simulink model "SG__MDL"  (R2022b)
settings: Solver=FixedStepAuto  StartTime=0.0  StopTime=Inf  FixedStep=ts  RelTol=1e-3  EnableMultiTasking=on
model workspace (MAT data in the model file):
  N_trig = Simulink.Parameter
  N_trig.Value = 4
  N_trig.Description = 'number of samples for triggered pulse for recording'
  N_trig.DataType = 'auto'
  N_trig.Complexity = 'real'
  N_trig.Dimensions = [1 1]
  Sig = Simulink.Signal
  Sig.DataType = 'auto'
  Sig.Dimensions = -1
  Sig.DimensionsMode = 'auto'
  Sig.Complexity = 'auto'
  Sig.SampleTime = -1
  Sig.SamplingMode = 'auto'
  dtf_a = Simulink.Parameter
  dtf_a.Value = [1  1  1; 1  1  1; 1  1  1; 1  1  1; 1  1  1; 1  1  1; 1  1  1; 1  1  1; 1  1  1; 1  1  1; 1  1  1; 1  1  1; 1  1  1; 1  1  1; 1  1  1; 1  1  1]
  dtf_a.DataType = 'auto'
  dtf_a.Complexity = 'real'
  dtf_a.Dimensions = [16 3]
  dtf_b = Simulink.Parameter
  dtf_b.Value = [0.5  0.5  0.5; 0.5  0.5  0.5; 0.5  0.5  0.5; 0.5  0.5  0.5; 0.5  0.5  0.5; 0.5  0.5  0.5; 0.5  0.5  0.5; 0.5  0.5  0.5; 0.5  0.5  0.5; 0.5  0.5  0.5; 0.5  0.5  0.5; 0.5  0.5  0.5; 0.5  0.5  0.5; 0.5  0.5  0.5; 0.5  0.5  0.5; 0.5  0.5  0.5]
  dtf_b.DataType = 'auto'
  dtf_b.Complexity = 'real'
  dtf_b.Dimensions = [16 3]
  enable_source = Simulink.Parameter
  enable_source.Value = 0
  enable_source.DataType = 'boolean'
  enable_source.Complexity = 'real'
  enable_source.Dimensions = [1 1]
  freq_fin = Simulink.Parameter
  freq_fin.Value = 1200
  freq_fin.DataType = 'auto'
  freq_fin.Complexity = 'real'
  freq_fin.Dimensions = [1 1]
  freq_ini = Simulink.Parameter
  freq_ini.Value = 150
  freq_ini.DataType = 'auto'
  freq_ini.Complexity = 'real'
  freq_ini.Dimensions = [1 1]
  k_L = Simulink.Parameter
  k_L.Value = [0; 0; 0; 0; 0; 0; 0; 0; 0; 0; 0; 0; 0; 0; 0; 0]
  k_L.Description = 'Coupling on left of ER. [Linear, NL]'
  k_L.DataType = 'auto'
  k_L.Complexity = 'real'
  k_L.Dimensions = [16 1]
  k_L_NL = Simulink.Parameter
  k_L_NL.Value = [0; 0; 0; 0; 0; 0; 0; 0; 0; 0; 0; 0; 0; 0; 0; 0]
  k_L_NL.Description = 'Coupling on left of ER. [Linear, NL]'
  k_L_NL.DataType = 'auto'
  k_L_NL.Complexity = 'real'
  k_L_NL.Dimensions = [16 1]
  k_O_NL = Simulink.Parameter
  k_O_NL.Value = [0; 0; 0; 0; 0; 0; 0; 0; 0; 0; 0; 0; 0; 0; 0; 0]
  k_O_NL.Description = 'Onsite nonlinearity'
  k_O_NL.DataType = 'auto'
  k_O_NL.Complexity = 'real'
  k_O_NL.Dimensions = [16 1]
  k_R = Simulink.Parameter
  k_R.Value = [0; 0; 0; 0; 0; 0; 0; 0; 0; 0; 0; 0; 0; 0; 0; 0]
  k_R.Description = 'Coupling on right of ER. [Linear, NL]'
  k_R.DataType = 'auto'
  k_R.Complexity = 'real'
  k_R.Dimensions = [16 1]
  k_R_NL = Simulink.Parameter
  k_R_NL.Value = [0; 0; 0; 0; 0; 0; 0; 0; 0; 0; 0; 0; 0; 0; 0; 0]
  k_R_NL.Description = 'Coupling on right of ER. [Linear, NL]'
  k_R_NL.DataType = 'auto'
  k_R_NL.Complexity = 'real'
  k_R_NL.Dimensions = [16 1]
  rec = Simulink.Parameter
  rec.Value = 1
  rec.DataType = 'boolean'
  rec.Complexity = 'real'
  rec.Dimensions = [1 1]
  src_select = Simulink.Parameter
  src_select.Value = 0
  src_select.DataType = 'auto'
  src_select.Complexity = 'real'
  src_select.Dimensions = [1 1]
  sweep_gain = Simulink.Parameter
  sweep_gain.Value = 0.02
  sweep_gain.DataType = 'auto'
  sweep_gain.Complexity = 'real'
  sweep_gain.Dimensions = [1 1]
  tmax = Simulink.Parameter
  tmax.Value = 10
  tmax.DataType = 'auto'
  tmax.Complexity = 'real'
  tmax.Dimensions = [1 1]
  ts_rec = Simulink.Parameter
  ts_rec.Value = 0.0001
  ts_rec.DataType = 'auto'
  ts_rec.Complexity = 'real'
  ts_rec.Dimensions = [1 1]
values from neighbouring files (symbols this model uses):
  ts = 400e-6    (= 0.0004)    [StartScript.m]
libraries: simulink x4, dspsrcs4 x2, hdlsllib x2, dspsigattribs x1, dspsigops x1, slrealtimeloglib x1
settings Model: SimulationMode=external  ExplicitPartitioning=on  DataflowThreadingImplementation=Pthreads  Creator=padlewsk  LastModifiedBy=padlewsk
settings SolverCC: AllowMultiTaskInputOutput=on  ConcurrentTasks=on  AlgebraicLoopSolver=TrustRegion  PositivePriorityOrder=on  AutoInsertRateTranBlk=on
settings DataIOCC: SaveFormat=StructureWithTime
settings OptimizationCC: GainParamInheritBuiltInType=on  RollThreshold=33  EfficientFloat2IntCast=on  SimCompilerOptimization=on
settings DebuggingCC: TasksWithSamePriorityMsg=none  UnconnectedInputMsg=warning  UnconnectedOutputMsg=warning  UnconnectedLineMsg=warning  ModelReferenceSymbolNameMessage=none
settings HardwareCC: ProdBitPerLong=64  ProdLongLongMode=on  ProdHWDeviceType=Intel->x86-64 (Linux 64)
settings ModelReferenceCC: EnableRefExpFcnMdlSchedulingChecks=on
settings RTWCC: Description=Simulink Real-Time  SystemTargetFile=slrealtime.tlc  TemplateMakefile=slrealtime_default_tmf  Toolchain=Simulink Real-Time Toolchain  BuildConfiguration=Faster Runs  CodeExecutionProfiling=on  TargetLang=C++
settings SimulinkRealTimeTargetCC: UseGCCFastMath=on

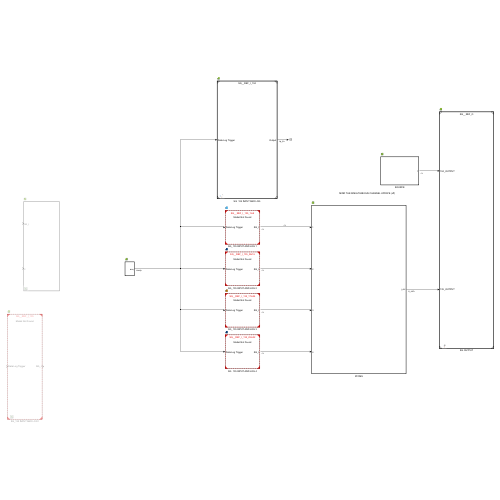
[thumbnail: Simulink's stored preview of the top-level diagram]
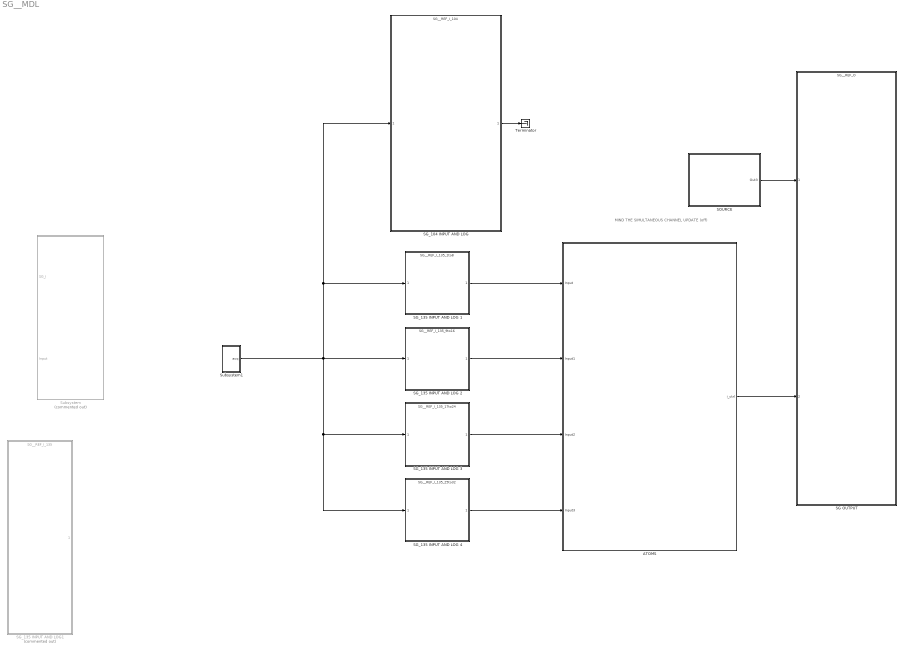
== system SG__MDL ==
  note: MIND THE SIMULTANEOUS CHANNEL UPDATE (off)
  ATOMS : Subsystem  TreatAsAtomicUnit=on
  SG OUTPUT : ModelReference  ModelNameDialog=SG__REF_O.slx  SimulationMode=Normal  ModelReferenceVersion=6.311
  SG_104 INPUT AND LOG : ModelReference  ModelNameDialog=SG__REF_I_104.slx  SimulationMode=Normal  ModelReferenceVersion=6.314
  SG_135 INPUT AND LOG 1 : ModelReference  ModelNameDialog=SG__REF_I_135_1to8.slx  SimulationMode=Normal  ModelReferenceVersion=6.293
  SG_135 INPUT AND LOG 2 : ModelReference  ModelNameDialog=SG__REF_I_135_9to16.slx  SimulationMode=Normal  ModelReferenceVersion=6.294
  SG_135 INPUT AND LOG 3 : ModelReference  ModelNameDialog=SG__REF_I_135_17to24.slx  SimulationMode=Normal  ModelReferenceVersion=6.296
  SG_135 INPUT AND LOG 4 : ModelReference  ModelNameDialog=SG__REF_I_135_25to32.slx  SimulationMode=Normal  ModelReferenceVersion=6.296
  SG_135 INPUT AND LOG1 : ModelReference  Commented=on  ModelNameDialog=SG__REF_I_135.slx  SimulationMode=Normal  ModelReferenceVersion=6.288
  SOURCE : Subsystem  TreatAsAtomicUnit=on
  Subsystem : Subsystem  Commented=on  TreatAsAtomicUnit=on
  Subsystem1 : Subsystem  TreatAsAtomicUnit=on
  Terminator : Terminator
  wires:
  SOURCE/1(Out3) -> SG OUTPUT/1
  SG_135 INPUT AND LOG 1/1 -> ATOMS/1(Input)
  ATOMS/1(i_ctrl) -> SG OUTPUT/2
  SG_104 INPUT AND LOG/1 -> Terminator/1
  Subsystem1/1(acq) -> SG_104 INPUT AND LOG/1, SG_135 INPUT AND LOG 1/1, SG_135 INPUT AND LOG 4/1, SG_135 INPUT AND LOG 3/1, SG_135 INPUT AND LOG 2/1
  SG_135 INPUT AND LOG 2/1 -> ATOMS/2(Input1)
  SG_135 INPUT AND LOG 3/1 -> ATOMS/3(Input2)
  SG_135 INPUT AND LOG 4/1 -> ATOMS/4(Input3)

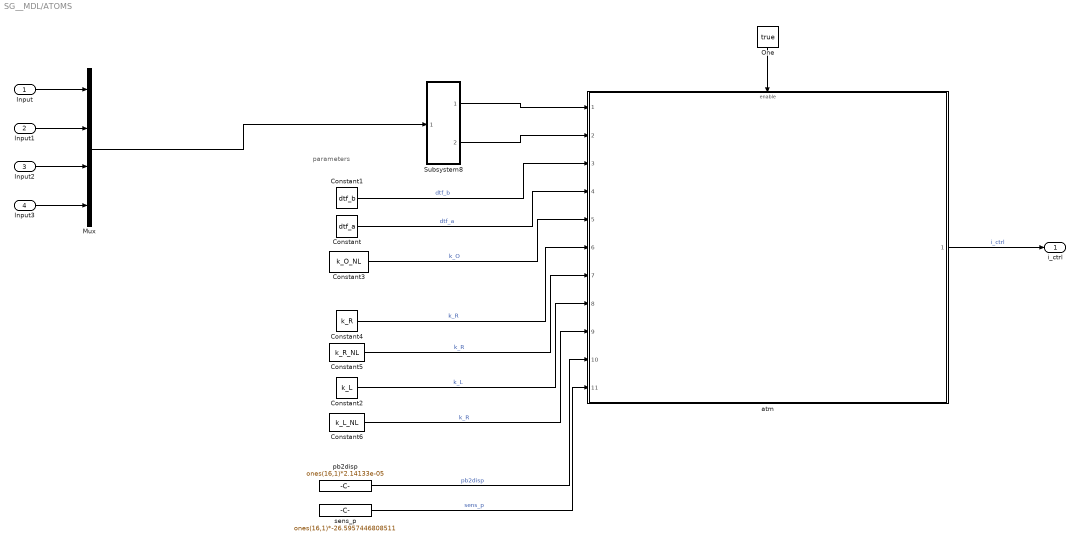
== system SG__MDL/ATOMS ==
  note: parameters
  Input : Inport
  Input1 : Inport  Port=2
  Input2 : Inport  Port=3
  Input3 : Inport  Port=4
  Constant : Constant  Value=dtf_a  SampleTime=-1
  Constant1 : Constant  Value=dtf_b  SampleTime=-1
  Constant2 : Constant  Value=k_L  SampleTime=-1
  Constant3 : Constant  Value=k_O_NL  SampleTime=-1
  Constant4 : Constant  Value=k_R  SampleTime=-1
  Constant5 : Constant  Value=k_R_NL  SampleTime=-1
  Constant6 : Constant  Value=k_L_NL  SampleTime=-1
  Mux : Mux
  One : Constant  Value=true  OutDataTypeStr=Inherit: Inherit via back propagation
  Subsystem8 : Subsystem
  atm : Subsystem  ReferencedSubsystem=atm
  pb2disp : Constant  Value=ones(16,1)*2.14133e-05  SampleTime=-1
  sens_p : Constant  Value=ones(16,1)*-26.5957446808511  SampleTime=-1
  i_ctrl : Outport
  wires:
  One/1 -> atm/Enable
  atm/1 -> i_ctrl/1  "i_ctrl"
  Constant1/1 -> atm/3  "dtf_b"
  Constant/1 -> atm/4  "dtf_a"
  Constant3/1 -> atm/5  "k_O"
  Constant4/1 -> atm/6  "k_R"
  Constant5/1 -> atm/7  "k_R"
  Constant2/1 -> atm/8  "k_L"
  Constant6/1 -> atm/9  "k_R"
  sens_p/1 -> atm/11  "sens_p"
  pb2disp/1 -> atm/10  "pb2disp"
  Subsystem8/2(Input1) -> atm/2
  Subsystem8/1(Input) -> atm/1
  Input/1 -> Mux/1
  Input1/1 -> Mux/2
  Input2/1 -> Mux/3
  Input3/1 -> Mux/4
  Mux/1 -> Subsystem8/1(SG_I)

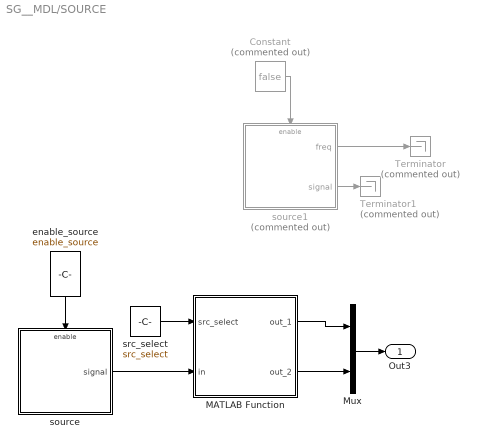
== system SG__MDL/SOURCE ==
  Constant : Constant  Commented=on  Value=false
  MATLAB Function : MATLAB Function  TreatAsAtomicUnit=on
  Mux : Mux  Inputs=2
  Terminator : Terminator  Commented=on
  Terminator1 : Terminator  Commented=on
  enable_source : Constant  Value=enable_source  SampleTime=-1
  source : Subsystem  TreatAsAtomicUnit=on
  source1 : Subsystem  Commented=on  TreatAsAtomicUnit=on
  src_select : Constant  Value=src_select
  Out3 : Outport
  wires:
  Mux/1 -> Out3/1
  Constant/1 -> source1/Enable
  source/1(signal) -> MATLAB Function/2(in)
  src_select/1 -> MATLAB Function/1(src_select)
  MATLAB Function/2(out_2) -> Mux/2
  enable_source/1 -> source/Enable
  source1/2(signal) -> Terminator1/1
  MATLAB Function/1(out_1) -> Mux/1
  source1/1(freq) -> Terminator/1

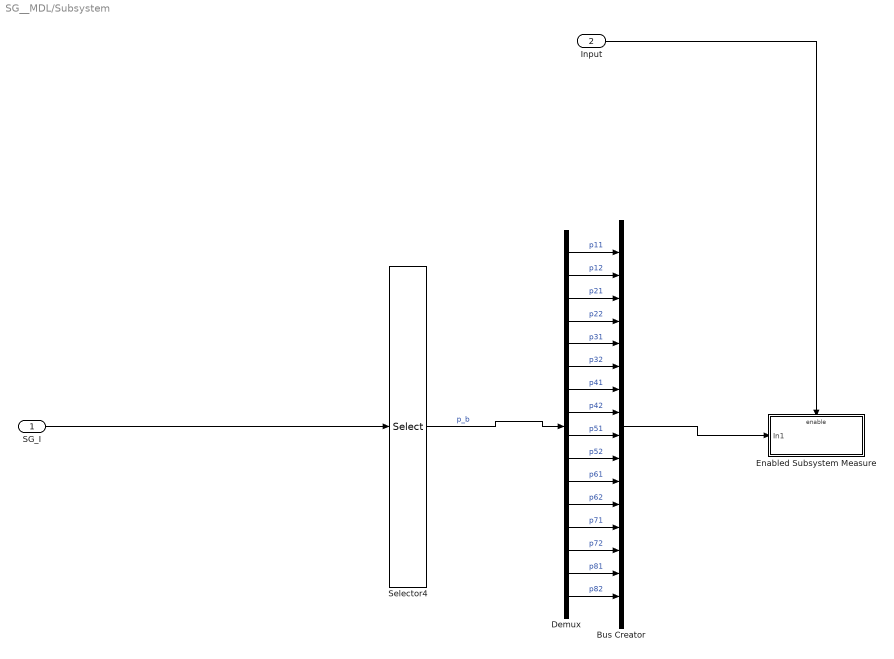
== system SG__MDL/Subsystem ==
  SG_I : Inport  SampleTime=ts
  Input : Inport  Port=2  OutDataTypeStr=boolean
  Bus Creator : BusCreator  Inputs=16
  Demux : Demux  Outputs=16
  Enabled Subsystem Measure : Subsystem
  Selector4 : Selector  InputPortWidth=32  IndexOptions=Index vector (dialog)  Indices=[1:2:32]  OutputSizes=1
  wires:
  Demux/15 -> Bus Creator/15  "p81"
  Bus Creator/1 -> Enabled Subsystem Measure/1(In1)
  Demux/9 -> Bus Creator/9  "p51"
  Demux/12 -> Bus Creator/12  "p62"
  Demux/1 -> Bus Creator/1  "p11"
  Demux/16 -> Bus Creator/16  "p82"
  Demux/8 -> Bus Creator/8  "p42"
  Demux/11 -> Bus Creator/11  "p61"
  Demux/2 -> Bus Creator/2  "p12"
  Demux/7 -> Bus Creator/7  "p41"
  Demux/10 -> Bus Creator/10  "p52"
  Demux/5 -> Bus Creator/5  "p31"
  Demux/13 -> Bus Creator/13  "p71"
  Demux/14 -> Bus Creator/14  "p72"
  Demux/4 -> Bus Creator/4  "p22"
  Demux/6 -> Bus Creator/6  "p32"
  Demux/3 -> Bus Creator/3  "p21"
  Selector4/1 -> Demux/1  "p_b"
  SG_I/1 -> Selector4/1
  Input/1 -> Enabled Subsystem Measure/Enable

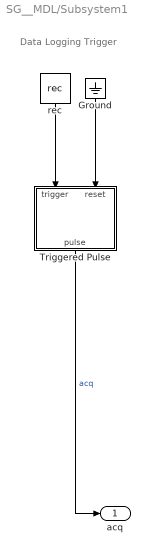
== system SG__MDL/Subsystem1 ==
  note: Data Logging Trigger
  Ground : Ground
  "Triggered Pulse " : Subsystem  TreatAsAtomicUnit=on  mask(Triggered Pulse){N=10/ts}
      mask prompts: N "Length (N samples)"
      mask help: Generates a single pulse of N samples length
  rec : Constant  Value=rec  SampleTime=-1
  acq : Outport  OutDataTypeStr=boolean
  wires:
  Ground/1 -> "Triggered Pulse "/2(reset)
  rec/1 -> "Triggered Pulse "/1(trigger)
  "Triggered Pulse "/1(pulse) -> acq/1  "acq"

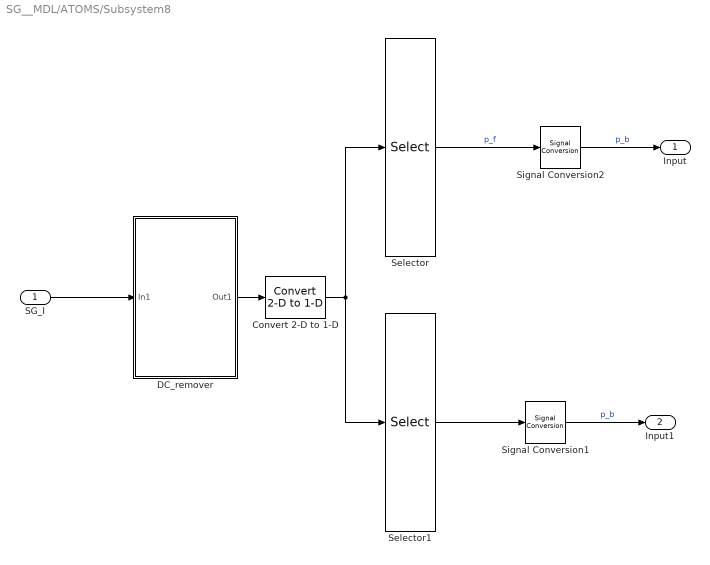
== system SG__MDL/ATOMS/Subsystem8 ==
  SG_I : Inport
  Convert 2-D to 1-D : dspsigattribs/Convert 2-D to 1-D
  DC_remover : Subsystem  TreatAsAtomicUnit=on
      settings: RTWSystemCode=Nonreusable function
  Selector : Selector  InputPortWidth=32  IndexOptions=Index vector (dialog)  Indices=1:2:32  OutputSizes=1
  Selector1 : Selector  InputPortWidth=32  IndexOptions=Index vector (dialog)  Indices=2:2:32  OutputSizes=1
  Signal Conversion1 : SignalConversion  OverrideOpt=off
  Signal Conversion2 : SignalConversion  OverrideOpt=off
  Input : Outport
  Input1 : Outport  Port=2
  wires:
  SG_I/1 -> DC_remover/1(In1)
  Selector1/1 -> Signal Conversion1/1
  DC_remover/1(Out1) -> Convert 2-D to 1-D/1
  Selector/1 -> Signal Conversion2/1  "p_f"
  Signal Conversion1/1 -> Input1/1  "p_b"
  Signal Conversion2/1 -> Input/1  "p_b"
  Convert 2-D to 1-D/1 -> Selector/1, Selector1/1

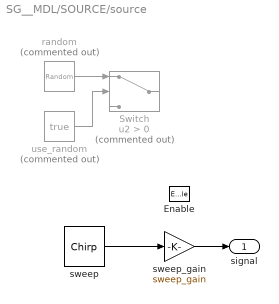
== system SG__MDL/SOURCE/source ==
  Enable : EnablePort  StatesWhenEnabling=reset
  Switch : Switch  Commented=on  Criteria=u2 > Threshold  SaturateOnIntegerOverflow=off  InputSameDT=off
  random : RandomNumber  Commented=on  Variance=0.5  SampleTime=3.5e-05
  sweep : dspsrcs4/Chirp  sweep=Logarithmic  mode=Bidirectional  f0=freq_ini  f1=freq_fin  t1=tmax*2  Tsweep=tmax*2  phase=0  Ts=ts_rec*0 + ts  spf=1  datatype=Double  OutputFrames=off
  sweep_gain : Gain  Gain=sweep_gain
  use_random : Constant  Commented=on  Value=true  SampleTime=-1
  signal : Outport  OutputWhenDisabled=reset  InitialOutput=0  VectorParamsAs1DForOutWhenUnconnected=off
  wires:
  use_random/1 -> Switch/2
  random/1 -> Switch/1
  sweep/1 -> sweep_gain/1
  sweep_gain/1 -> signal/1

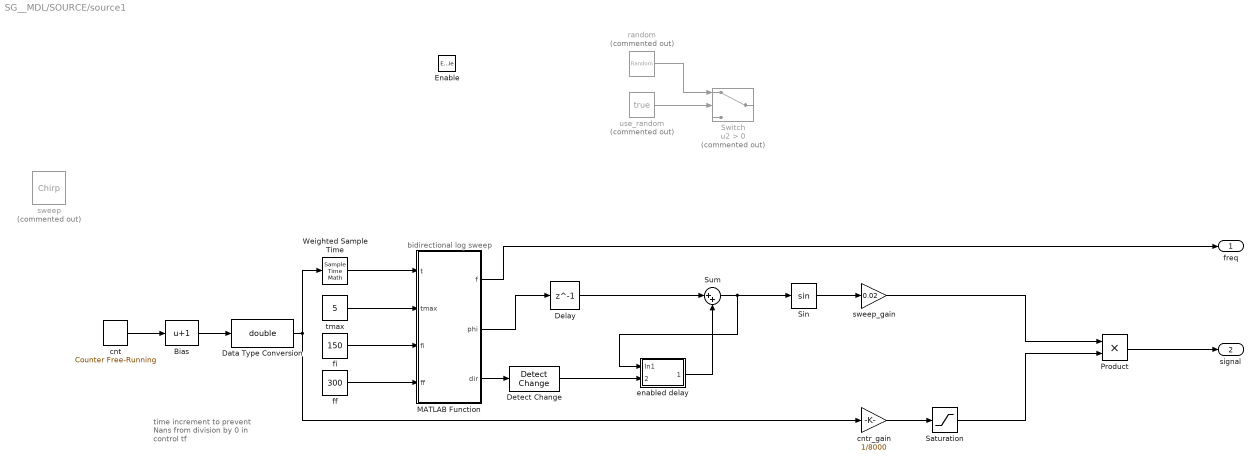
== system SG__MDL/SOURCE/source1 ==
  note: bidirectional log sweep
  note: time increment to prevent Nans from division by 0 in control tf
  Enable : EnablePort  StatesWhenEnabling=reset
  Bias : Bias  Bias=1  SaturateOnIntegerOverflow=off
  Data Type Conversion : DataTypeConversion  OutDataTypeStr=double  SaturateOnIntegerOverflow=off  RndMeth=Floor
  Delay : Delay  DelayLength=1
  Detect Change : simulink/Logic and Bit Operations/Detect Change  vinit=false  OutDataTypeStr=boolean
  MATLAB Function : MATLAB Function  TreatAsAtomicUnit=on
  Product : Product
  Saturation : Saturate  UpperLimit=1  LowerLimit=0
  Sin : Trigonometry
  Sum : Sum  Inputs=|++
  Switch : Switch  Commented=on  Criteria=u2 > Threshold  SaturateOnIntegerOverflow=off  InputSameDT=off
  Weighted Sample Time : SampleTimeMath  TsampMathOp=*
  cnt : simulink/Sources/Counter Free-Running  NumBits=32  tsamp=-1
  cntr_gain : Gain  Gain=1/8000  ParamDataTypeStr=double
  enabled delay : Subsystem
  ff : Constant  Value=300
  fi : Constant  Value=150
  random : RandomNumber  Commented=on  Variance=0.5  SampleTime=3.5e-05
  sweep : dspsrcs4/Chirp  Commented=on  sweep=Logarithmic  mode=Bidirectional  f0=150  f1=1200  t1=10  Tsweep=20  phase=0  Ts=3.5e-05  spf=1  datatype=Double  OutputFrames=off
  sweep_gain : Gain  Gain=0.02
  tmax : Constant  Value=5
  use_random : Constant  Commented=on  Value=true  SampleTime=-1
  freq : Outport  OutputWhenDisabled=reset  InitialOutput=0  VectorParamsAs1DForOutWhenUnconnected=off
  signal : Outport  Port=2  OutputWhenDisabled=reset  InitialOutput=0  VectorParamsAs1DForOutWhenUnconnected=off
  wires:
  use_random/1 -> Switch/2
  random/1 -> Switch/1
  sweep_gain/1 -> Product/1
  cntr_gain/1 -> Saturation/1
  Product/1 -> signal/1
  MATLAB Function/2(phi) -> Delay/1
  Saturation/1 -> Product/2
  Weighted Sample Time/1 -> MATLAB Function/1(t)
  Data Type Conversion/1 -> cntr_gain/1, Weighted Sample Time/1
  MATLAB Function/1(f) -> freq/1
  Sin/1 -> sweep_gain/1
  MATLAB Function/3(dir) -> Detect Change/1
  Detect Change/1 -> enabled delay/2(enable)
  Delay/1 -> Sum/1
  enabled delay/1(Out1) -> Sum/2
  Sum/1 -> enabled delay/1(In1), Sin/1
  cnt/1 -> Bias/1
  Bias/1 -> Data Type Conversion/1
  ff/1 -> MATLAB Function/4(ff)
  tmax/1 -> MATLAB Function/2(tmax)
  fi/1 -> MATLAB Function/3(fi)

== system SG__MDL/Subsystem/Enabled Subsystem Measure ==
  In1 : Inport
  Enable : EnablePort
  File Log : slrealtimeloglib/File Log  decimation=1  inputProcessing=Elements as channels (sample based)
  wires:
  In1/1 -> File Log/1

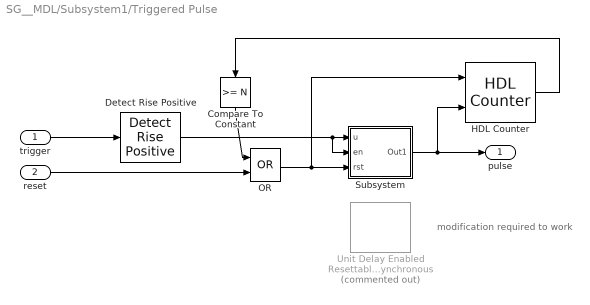
== system SG__MDL/Subsystem1/Triggered Pulse  ==
  note: modification required to work
  trigger : Inport
  reset : Inport  Port=2
  Compare To Constant : simulink/Logic and Bit Operations/Compare To Constant  relop=>=  const=N  OutDataTypeStr=boolean
  Detect Rise Positive : simulink/Logic and Bit Operations/Detect Rise Positive  vinit=0  OutDataTypeStr=boolean
  HDL Counter : hdlsllib/Sources/HDL Counter  CountType=Free running  CountInit=1  CountStep=1  CountMax=25  CountFromType=Initial value  CountFrom=1  CountResetPort=on  CountLoadPort=off  CountEnbPort=on  CountDirPort=off  CountHitOutputPort=off  CountDataType=Unsigned  CountWordLen=32  CountFracLen=0  CountSampTime=1
  OR : Logic  Operator=OR  AllPortsSameDT=off  OutDataTypeStr=boolean
  Subsystem : Subsystem
  Unit Delay Enabled Resettable Synchronous : hdlsllib/Discrete/Unit Delay Enabled Resettable Synchronous  Commented=on  InitialCondition=0.0  SampleTime=-1
  pulse : Outport  VectorParamsAs1DForOutWhenUnconnected=off
  wires:
  OR/1 -> Subsystem/3(rst), HDL Counter/1
  trigger/1 -> Detect Rise Positive/1
  Subsystem/1(Out1) -> HDL Counter/2, pulse/1
  Compare To Constant/1 -> OR/1
  reset/1 -> OR/2
  Detect Rise Positive/1 -> Subsystem/2(en), Subsystem/1(u)
  HDL Counter/1 -> Compare To Constant/1

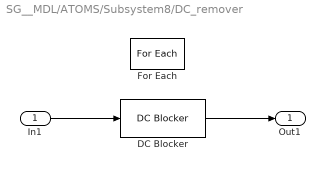
== system SG__MDL/ATOMS/Subsystem8/DC_remover ==
  In1 : Inport  Partition=on  PartitionDimension=1  PartitionWidth=1  PartitionOffset=0
  DC Blocker : dspsigops/DC Blocker  Algorithm=FIR  NormalizedBandwidth=0.001  Length=20  Order=6  SimulateUsing=Code generation
      settings: LibrarySourceBlock=dsphdlsupportsigops/DC Blocker
  For Each : ForEach  DisableCoverage=on
  Out1 : Outport  ConcatenationDimension=1
  wires:
  In1/1 -> DC Blocker/1
  DC Blocker/1 -> Out1/1

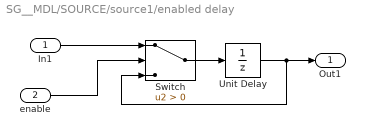
== system SG__MDL/SOURCE/source1/enabled delay ==
  In1 : Inport
  enable : Inport  Port=2
  Switch : Switch  Criteria=u2 > Threshold  SaturateOnIntegerOverflow=off  InputSameDT=off
  Unit Delay : UnitDelay  SampleTime=-1  HasFrameUpgradeWarning=on
  Out1 : Outport
  wires:
  Unit Delay/1 -> Switch/3, Out1/1
  Switch/1 -> Unit Delay/1
  In1/1 -> Switch/1
  enable/1 -> Switch/2

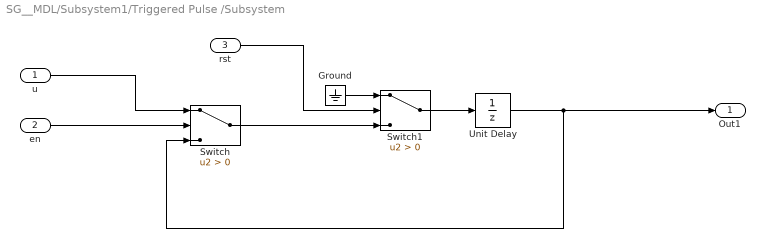
== system SG__MDL/Subsystem1/Triggered Pulse /Subsystem ==
  u : Inport
  en : Inport  Port=2
  rst : Inport  Port=3
  Ground : Ground
  Switch : Switch  Criteria=u2 > Threshold  SaturateOnIntegerOverflow=off  InputSameDT=off
  Switch1 : Switch  Criteria=u2 > Threshold  SaturateOnIntegerOverflow=off  InputSameDT=off
  Unit Delay : UnitDelay  SampleTime=-1  HasFrameUpgradeWarning=on
  Out1 : Outport
  wires:
  Unit Delay/1 -> Switch/3, Out1/1
  en/1 -> Switch/2
  u/1 -> Switch/1
  rst/1 -> Switch1/2
  Ground/1 -> Switch1/1
  Switch1/1 -> Unit Delay/1
  Switch/1 -> Switch1/3

== matlab function SG__MDL/SOURCE/source1/MATLAB Function ==
  data: f output; t input; tmax input; phi output; dir output; fi input; ff input
function [f, phi, dir] = fcn(t, tmax, fi, ff)
%tmax is the time at which the maximum frequency is reached

t = mod(t, 2*tmax);

if t < tmax
    % up
    dir = 1;
    
    
    % linear (CF wikipedia)
%     phi = 2*pi*(0.5*(ff - fi)*t^2/tmax + fi*t);
%     f = fi + (ff - fi)*t/tmax;
    
    % logarithmic %%% https://en.wikipedia.org/wiki/Chirp
    k = log((ff/fi)^(1/tmax));
    phi = 2*pi*fi*(exp(k*t) - 1)/k;
    f = fi*exp(k*t);
else
    % down
    dir = -1;
    
    
    % linear (CF wikipedia)
%     phi = 2*pi*(0.5*(fi - ff)*(t-tmax)^2/tmax + ff*(t-tmax)); % linear
%     f = ff + (fi - ff)*(t - tmax)/tmax;
    
    % logarithmic
    k = log((fi/ff)^(1/tmax));
    phi = 2*pi*ff*(exp(k*(t - tmax)) - 1)/k;
    f = ff*exp(k*(t-tmax));
end

phi = mod(phi, 2*pi);

== matlab function SG__MDL/SOURCE/MATLAB Function ==
  data: src_select input; in input; out_1 output; out_2 output
function [out_1, out_2] = fct(src_select, in)
out_1 = 0;
out_2 = 0;
if src_select == 1
    out_1 = in;
elseif src_select == 2
    out_2 = in;
end
